simulink model "RobotControl1_640_480"  (R2015a)
settings: Solver=ode3  StartTime=0.0  StopTime=inf  FixedStep=1/30  RelTol=1e-3
undefined symbols (not defined in the file or in its folder): RGB24
libraries: xpcutilitieslib x31, slrtlib x8, AAxpcseriallibold x7, xpcobsoletelib x5, xpcvideousblib x3, dspstat3 x1, simulink x1
settings Model: SimulationMode=external  Creator=farbod  LastModifiedBy=sd0016
settings SolverCC: EnableConcurrentExecution=on
settings DataIOCC: SignalLoggingSaveFormat=ModelDataLogs
settings OptimizationCC: BlockReduction=off  OptimizeBlockIOStorage=off  BufferReuse=off  GlobalBufferReuse=off  ExpressionFolding=off  ExpressionDepthLimit=2147483647  LocalBlockOutputs=off
settings DebuggingCC: UnderspecifiedInitializationDetection=Classic  MergeDetectMultiDrivingBlocksExec=none  FcnCallInpInsideContextMsg=UseLocalSettings  StateNameClashWarn=warning
settings HardwareCC: ProdIntDivRoundTo=Zero  ProdEndianess=LittleEndian  ProdLongLongMode=on  ProdHWDeviceType=Generic->32-bit x86 compatible  TargetBitPerLong=64  TargetBitPerPointer=64  TargetIntDivRoundTo=Zero  TargetEndianess=LittleEndian  TargetWordSize=64  TargetHWDeviceType=Intel->x86-64
settings SFSimCC: SimParseCustomCode=off
settings RTWCC: SystemTargetFile=slrt.tlc  TemplateMakefile=slrt_default_tmf  Description=Simulink Real-Time  RTWVerbose=off  RTWCompilerOptimization=on
settings CodeAppCC: MaxIdLength=95
settings SimulinkRealTimeCC: GeneratePreprocessorConditionals=Disable all

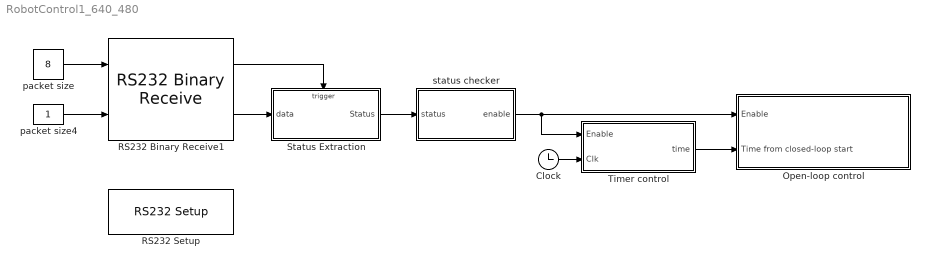
== system RobotControl1_640_480 ==
  Clock : Clock
  Open-loop control : Subsystem
  RS232 Binary Receive1 : AAxpcseriallibold/Obsolete/Binary Mode/RS232 Binary Receive  port=COM1  width=8  samptime=-1
  "RS232 Setup " : AAxpcseriallibold/Obsolete/RS232 Setup   port=COM1  baud=115200  dbits=8  sbits=1  parity=None  prot=None  sbuf=2048  rbuf=2048  initstruct=[]  termstruct=[]
  Status Extraction : Subsystem  TreatAsAtomicUnit=on
  Timer control : Subsystem
  packet size : Constant  Value=8
  packet size4 : Constant
  status checker : MATLAB Function  TreatAsAtomicUnit=on
  wires:
  status checker/1(enable) -> Open-loop control/1("Enable "), Timer control/1(Enable)
  Status Extraction/1(Status) -> status checker/1(status)
  RS232 Binary Receive1/2 -> Status Extraction/1(data)
  RS232 Binary Receive1/1 -> Status Extraction/Trigger
  packet size4/1 -> RS232 Binary Receive1/2
  packet size/1 -> RS232 Binary Receive1/1
  Timer control/1(time) -> Open-loop control/2(Time from closed-loop start)
  Clock/1 -> Timer control/2(Clk)

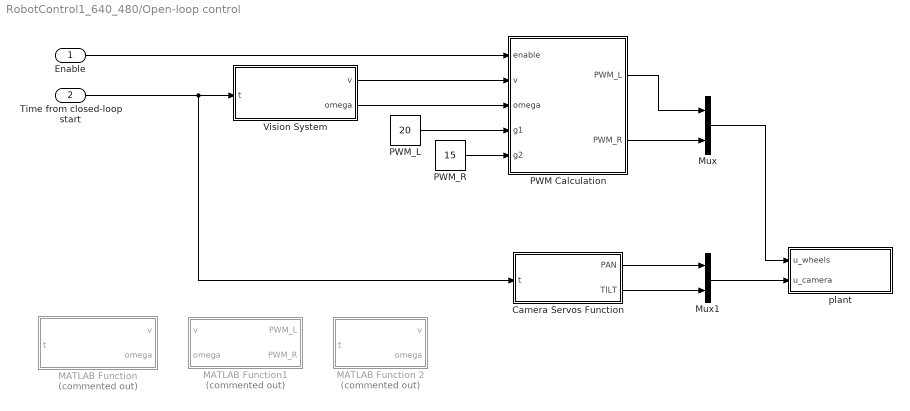
== system RobotControl1_640_480/Open-loop control ==
  "Enable " : Inport
  Time from closed-loop start : Inport  Port=2
  " MATLAB Function1" : MATLAB Function  Commented=on  TreatAsAtomicUnit=on
  Camera Servos Function : MATLAB Function  TreatAsAtomicUnit=on
  MATLAB Function : MATLAB Function  Commented=on  TreatAsAtomicUnit=on
  MATLAB Function 2 : MATLAB Function  Commented=on  TreatAsAtomicUnit=on
  Mux : Mux  Inputs=2
  Mux1 : Mux  Inputs=2
  PWM Calculation : MATLAB Function  TreatAsAtomicUnit=on
  PWM_L : Constant  Value=20
  PWM_R : Constant  Value=15
  Vision System : Subsystem
  plant : Subsystem
  wires:
  Mux/1 -> plant/1(u_wheels)
  Camera Servos Function/1(PAN) -> Mux1/1
  Camera Servos Function/2(TILT) -> Mux1/2
  Mux1/1 -> plant/2(u_camera)
  PWM Calculation/2(PWM_R) -> Mux/2
  "Enable "/1 -> PWM Calculation/1(enable)
  PWM Calculation/1(PWM_L) -> Mux/1
  Time from closed-loop start/1 -> Camera Servos Function/1(t), Vision System/1(t)
  Vision System/1(v) -> PWM Calculation/2(v)
  Vision System/2(omega) -> PWM Calculation/3(omega)
  PWM_L/1 -> PWM Calculation/4(g1)
  PWM_R/1 -> PWM Calculation/5(g2)

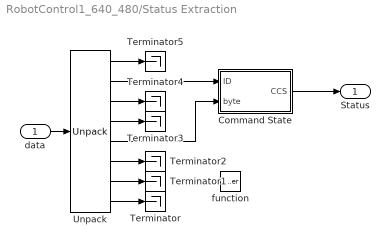
== system RobotControl1_640_480/Status Extraction ==
  data : Inport
  function : TriggerPort  TriggerType=function-call  OutputDataType=int8
  Command State : MATLAB Function  TreatAsAtomicUnit=on
  Terminator{,1..5} (6 alike) : Terminator
  Unpack : xpcobsoletelib/Utilities/Unpack   dimensions={1,1,1,1,1,1,1,1}  datatypes={'uint8','uint8','uint8','uint8','uint8','uint8','uint8','uint8'}  byteAlign=1
  Status : Outport
  wires:
  data/1 -> Unpack/1
  Command State/1(CCS) -> Status/1
  Unpack/5 -> Command State/2(byte)
  Unpack/2 -> Command State/1(ID)
  Unpack/8 -> Terminator/1
  Unpack/1 -> Terminator5/1
  Unpack/3 -> Terminator4/1
  Unpack/4 -> Terminator3/1
  Unpack/6 -> Terminator2/1
  Unpack/7 -> Terminator1/1

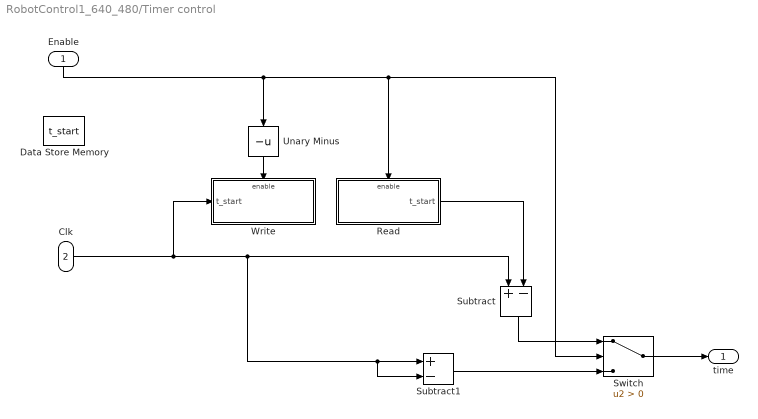
== system RobotControl1_640_480/Timer control ==
  Enable : Inport
  Clk : Inport  Port=2
  Data Store Memory : DataStoreMemory  DataStoreName=t_start  ReadBeforeWriteMsg=warning  WriteAfterWriteMsg=warning  WriteAfterReadMsg=warning
  Read : Subsystem  TreatAsAtomicUnit=on
  Subtract : Sum  Inputs=+-
  Subtract1 : Sum  Inputs=+-
  Switch : Switch  Criteria=u2 > Threshold
  Unary Minus : UnaryMinus
  Write : Subsystem  TreatAsAtomicUnit=on
  time : Outport
  wires:
  Read/1(t_start) -> Subtract/2
  Clk/1 -> Write/1(t_start), Subtract1/2, Subtract1/1, Subtract/1
  Unary Minus/1 -> Write/Enable
  Enable/1 -> Unary Minus/1, Read/Enable, Switch/2
  Switch/1 -> time/1
  Subtract/1 -> Switch/1
  Subtract1/1 -> Switch/3

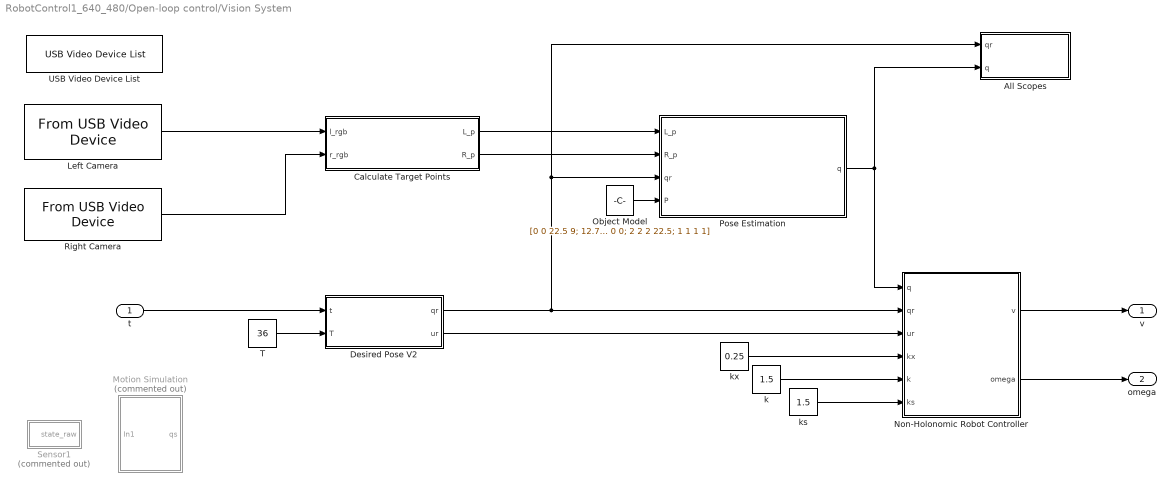
== system RobotControl1_640_480/Open-loop control/Vision System ==
  t : Inport
  All Scopes : Subsystem
  Calculate Target Points : MATLAB Function  TreatAsAtomicUnit=on
  Desired Pose V2 : MATLAB Function  TreatAsAtomicUnit=on
  Left Camera : xpcvideousblib/From USB Video Device  sconf=<Select a configuration>  paddr=1.0  iwidth=640  iheight=480  fint=1/30  ffmt=Uncompressed  cfmt=RGB24 (8:8:8)  isig=One multidimensional signal  trigger=off  status=off  updateBlock=1
  Motion Simulation : Subsystem  Commented=on
  Non-Holonomic Robot Controller : MATLAB Function  TreatAsAtomicUnit=on
  Object Model : Constant  Value=[0 0 22.5 9; 12.75 -12.75 0 0; 2 2 2 22.5; 1 1 1 1]
  Pose Estimation : MATLAB Function  TreatAsAtomicUnit=on
  Right Camera : xpcvideousblib/From USB Video Device  sconf=<Select a configuration>  paddr=1.3  iwidth=640  iheight=480  fint=1/30  ffmt=Uncompressed  cfmt=RGB24 (8:8:8)  isig=One multidimensional signal  trigger=off  status=off  updateBlock=1
  Sensor1 : Subsystem  Commented=on
  T : Constant  Value=36
  USB Video Device List : xpcvideousblib/USB Video Device List  usb_search=on  ShowInLibBrowser=0
  k : Constant  Value=1.5
  ks : Constant  Value=1.5
  kx : Constant  Value=0.25
  v : Outport
  omega : Outport  Port=2
  wires:
  Non-Holonomic Robot Controller/1(v) -> v/1
  Non-Holonomic Robot Controller/2(omega) -> omega/1
  Object Model/1 -> Pose Estimation/4(P)
  Left Camera/1 -> Calculate Target Points/1(l_rgb)
  Right Camera/1 -> Calculate Target Points/2(r_rgb)
  Calculate Target Points/1(L_p) -> Pose Estimation/1(L_p)
  Calculate Target Points/2(R_p) -> Pose Estimation/2(R_p)
  Desired Pose V2/1(qr) -> Pose Estimation/3(qr), All Scopes/1(qr), Non-Holonomic Robot Controller/2(qr)
  Desired Pose V2/2(ur) -> Non-Holonomic Robot Controller/3(ur)
  k/1 -> Non-Holonomic Robot Controller/5(k)
  kx/1 -> Non-Holonomic Robot Controller/4(kx)
  ks/1 -> Non-Holonomic Robot Controller/6(ks)
  T/1 -> Desired Pose V2/2(T)
  t/1 -> Desired Pose V2/1(t)
  Pose Estimation/1(q) -> All Scopes/2(q), Non-Holonomic Robot Controller/1(q)

== system RobotControl1_640_480/Open-loop control/plant ==
  u_wheels : Inport
  u_camera : Inport  Port=2
  Demux : Demux  Outputs=2
  Demux1 : Demux  Outputs=2
  Send Serial Packet to Servo Controller And recieve status message from SSC : Subsystem  TreatAsAtomicUnit=on
  Servo1 : Constant  Value=1500  OutDataTypeStr=uint16
  pulse transformer camera : MATLAB Function  TreatAsAtomicUnit=on
  pulse transformer1 : MATLAB Function  TreatAsAtomicUnit=on
  wires:
  Servo1/1 -> Send Serial Packet to Servo Controller And recieve status message from SSC/6(Servo6), Send Serial Packet to Servo Controller And recieve status message from SSC/8(Servo8), Send Serial Packet to Servo Controller And recieve status message from SSC/4(Servo4), Send Serial Packet to Servo Controller And recieve status message from SSC/1(Servo1)
  u_wheels/1 -> Demux/1
  Demux/1 -> pulse transformer1/1(Left_PWM_I)
  Demux/2 -> pulse transformer1/2(Right_PWM_I)
  u_camera/1 -> Demux1/1
  pulse transformer1/1(Left_PWM) -> Send Serial Packet to Servo Controller And recieve status message from SSC/2(Left)
  pulse transformer1/2(Right_PWM) -> Send Serial Packet to Servo Controller And recieve status message from SSC/3(Right)
  Demux1/1 -> pulse transformer camera/1(PAN)
  Demux1/2 -> pulse transformer camera/2(TILT)
  pulse transformer camera/1(PAN_O) -> Send Serial Packet to Servo Controller And recieve status message from SSC/5(Pan)
  pulse transformer camera/2(TILT_O) -> Send Serial Packet to Servo Controller And recieve status message from SSC/7(Tilt)

== system RobotControl1_640_480/Timer control/Read ==
  Enable : EnablePort
  Data Store Read : DataStoreRead  DataStoreName=t_start
  t_start : Outport
  wires:
  Data Store Read/1 -> t_start/1

== system RobotControl1_640_480/Timer control/Write ==
  t_start : Inport
  Enable : EnablePort
  Data Store Write : DataStoreWrite  DataStoreName=t_start
  wires:
  t_start/1 -> Data Store Write/1

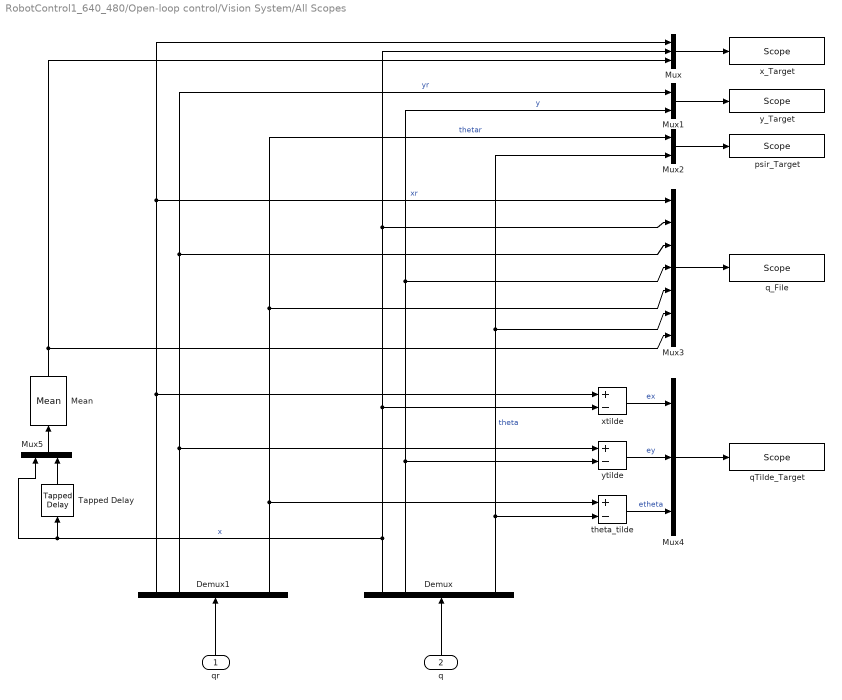
== system RobotControl1_640_480/Open-loop control/Vision System/All Scopes ==
  qr : Inport
  q : Inport  Port=2
  Demux : Demux  Outputs=6
  Demux1 : Demux  Outputs=6
  Mean : dspstat3/Mean  run=off  reset_popup=None  InputProcessing=Columns as channels (frame based)  directionMode=Each column  dimension=1  treatSBRowAsCol=off  roiEnable=off  roiType=Rectangles  roiPortion=Entire ROI  roiOutput=Individual statistics for each ROI  roiFlag=off  outputDataTypeStr=Inherit: Same as accumulator  outputLastDataTypeStr=Inherit: Same as accumulator  outputMin=[]  outputMax=[]  roundingMode=Floor  overflowMode=off
  Mux : Mux  Inputs=3
  Mux1 : Mux  Inputs=2
  Mux2 : Mux  Inputs=2
  Mux3 : Mux  Inputs=7
  Mux4 : Mux  Inputs=3
  Mux5 : Mux  Inputs=2
  Tapped Delay : simulink/Discrete/Tapped Delay  vinit=[0 0]  samptime=-1  NumDelays=2  DelayOrder=Oldest  includeCurrent=off
  "psir_Target " : slrtlib/Displays and Logging/Scope   scopeno=6  scopetype=Target  autostart=on  viewmode=Graphical rolling  formatstr='%15.6f'  grid=on  ylimits=[-3, 3]  nosamples=1000  noprepostsamples=0  interleave=1  triggermode=FreeRun  triggersignal=1  trigsignalfromport=off  triggerlevel=0.0  triggerslope=Either  triggerscope=1  triggersample=0  filename=data.dat  mode=Lazy  writesize=512  autorestart=off  dynamicfilemode=off  maxwritefilesize=512*1024^2
  qTilde_Target : slrtlib/Displays and Logging/Scope   scopeno=3  scopetype=Target  autostart=on  viewmode=Numerical  formatstr='%15.6f'  grid=on  ylimits=[0,0]  nosamples=3  noprepostsamples=0  interleave=1  triggermode=FreeRun  triggersignal=1  trigsignalfromport=off  triggerlevel=0.0  triggerslope=Either  triggerscope=1  triggersample=0  filename=data.dat  mode=Lazy  writesize=512  autorestart=off  dynamicfilemode=off  maxwritefilesize=512*1024^2
  q_File : slrtlib/Displays and Logging/Scope   scopeno=2  scopetype=File  autostart=on  viewmode=Graphical redraw  formatstr='%15.6f'  grid=on  ylimits=[0,0]  nosamples=6000  noprepostsamples=0  interleave=1  triggermode=FreeRun  triggersignal=1  trigsignalfromport=off  triggerlevel=0.0  triggerslope=Either  triggerscope=1  triggersample=0  filename=q.dat  mode=Lazy  writesize=512  autorestart=off  dynamicfilemode=off  maxwritefilesize=512*1024^2
  theta_tilde : Sum  Inputs=+-
  "x_Target " : slrtlib/Displays and Logging/Scope   scopeno=1  scopetype=Target  autostart=on  viewmode=Graphical rolling  formatstr='%15.6f'  grid=on  ylimits=[-4.5, 0.5]  nosamples=1000  noprepostsamples=0  interleave=1  triggermode=FreeRun  triggersignal=1  trigsignalfromport=off  triggerlevel=0.0  triggerslope=Either  triggerscope=1  triggersample=0  filename=data.dat  mode=Lazy  writesize=512  autorestart=off  dynamicfilemode=off  maxwritefilesize=512*1024^2
  xtilde : Sum  Inputs=+-
  y_Target : slrtlib/Displays and Logging/Scope   scopeno=4  scopetype=Target  autostart=on  viewmode=Graphical rolling  formatstr='%15.6f'  grid=on  ylimits=[-2,2]  nosamples=1000  noprepostsamples=0  interleave=1  triggermode=FreeRun  triggersignal=1  trigsignalfromport=off  triggerlevel=0.0  triggerslope=Either  triggerscope=1  triggersample=0  filename=data.dat  mode=Lazy  writesize=512  autorestart=off  dynamicfilemode=off  maxwritefilesize=512*1024^2
  ytilde : Sum  Inputs=+-
  wires:
  q/1 -> Demux/1
  Demux1/1 -> xtilde/1, Mux/1, Mux3/1  "xr"
  Demux1/2 -> ytilde/1, Mux1/1, Mux3/3  "yr"
  Mux3/1 -> q_File/1
  qr/1 -> Demux1/1
  Mux1/1 -> y_Target/1
  Mux/1 -> "x_Target "/1
  Mux2/1 -> "psir_Target "/1
  Demux/6 -> theta_tilde/2, Mux3/6, Mux2/2  "theta"
  Demux1/6 -> theta_tilde/1, Mux2/1, Mux3/5  "thetar"
  Demux/2 -> ytilde/2, Mux3/4, Mux1/2  "y"
  Demux/1 -> Mux5/1, Tapped Delay/1, xtilde/2, Mux3/2, Mux/2  "x"
  theta_tilde/1 -> Mux4/3  "etheta"
  ytilde/1 -> Mux4/2  "ey"
  xtilde/1 -> Mux4/1  "ex"
  Mux4/1 -> qTilde_Target/1
  Tapped Delay/1 -> Mux5/2
  Mean/1 -> Mux/3, Mux3/7
  Mux5/1 -> Mean/1

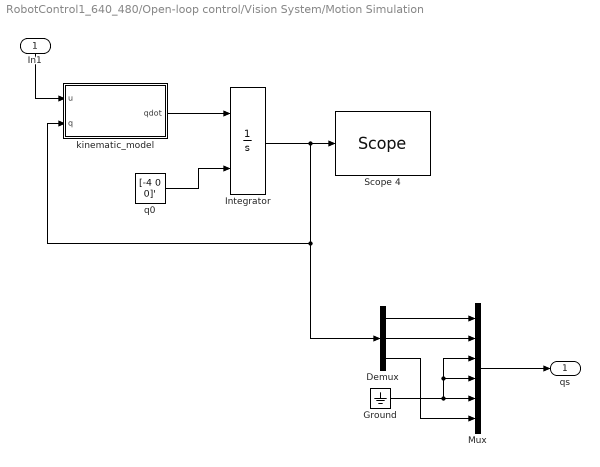
== system RobotControl1_640_480/Open-loop control/Vision System/Motion Simulation ==
  In1 : Inport
  Demux : Demux  Outputs=3
  Ground : Ground
  Integrator : Integrator  InitialConditionSource=external
  Mux : Mux  Inputs=6
  Scope 4 : slrtlib/Displays and Logging/Scope   scopeno=30  scopetype=File  autostart=on  viewmode=Graphical rolling  formatstr='%15.6f'  grid=on  ylimits=[0,0]  nosamples=250  noprepostsamples=0  interleave=1  triggermode=FreeRun  triggersignal=1  trigsignalfromport=off  triggerlevel=0.0  triggerslope=Either  triggerscope=1  triggersample=0  filename=data.dat  mode=Lazy  writesize=512  autorestart=off  dynamicfilemode=off  maxwritefilesize=512*1024^2
  kinematic_model : MATLAB Function  TreatAsAtomicUnit=on
  q0 : Constant  Value=[-4 0 0]'
  qs : Outport
  wires:
  kinematic_model/1(qdot) -> Integrator/1
  In1/1 -> kinematic_model/1(u)
  Integrator/1 -> Demux/1, kinematic_model/2(q), Scope 4/1
  q0/1 -> Integrator/2
  Mux/1 -> qs/1
  Demux/1 -> Mux/1
  Demux/2 -> Mux/2
  Demux/3 -> Mux/6
  Ground/1 -> Mux/5, Mux/3, Mux/4

== system RobotControl1_640_480/Open-loop control/Vision System/Sensor1 ==
  Add : Sum  Inputs=+-
  Clock2 : Clock
  Command State : MATLAB Function  TreatAsAtomicUnit=on
  IMU Trigger : Subsystem
  Read_Filter_ConvertTo2D : Subsystem
  delay : Constant
  state_raw : Outport
  wires:
  Clock2/1 -> Add/1, Command State/1(clock)
  Read_Filter_ConvertTo2D/1(state_raw) -> state_raw/1
  delay/1 -> Add/2
  Add/1 -> Read_Filter_ConvertTo2D/Enable
  Command State/1(Status) -> IMU Trigger/Enable

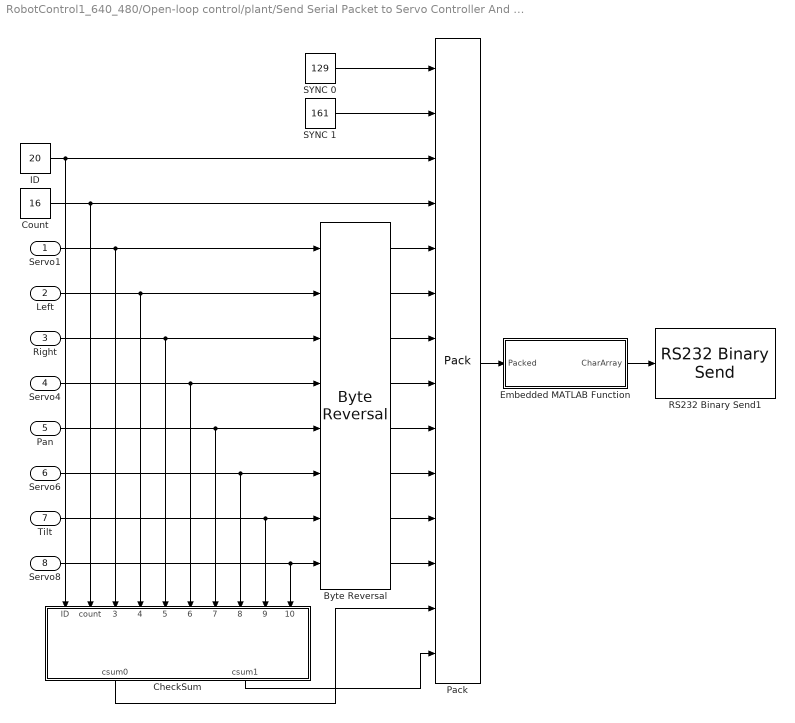
== system RobotControl1_640_480/Open-loop control/plant/Send Serial Packet to Servo Controller And recieve status message from SSC ==
  Servo1 : Inport  OutDataTypeStr=uint16
  Left : Inport  Port=2  OutDataTypeStr=uint16
  Right : Inport  Port=3  OutDataTypeStr=uint16
  Servo4 : Inport  Port=4  OutDataTypeStr=uint16
  Pan : Inport  Port=5  OutDataTypeStr=uint16
  Servo6 : Inport  Port=6  OutDataTypeStr=uint16
  Tilt : Inport  Port=7  OutDataTypeStr=uint16
  Servo8 : Inport  Port=8  OutDataTypeStr=uint16
  Byte Reversal : xpcutilitieslib/Byte Reversal   numInp=8
  CheckSum : MATLAB Function  TreatAsAtomicUnit=on
  Count : Constant  Value=16  OutDataTypeStr=uint8
  Embedded MATLAB Function : MATLAB Function  TreatAsAtomicUnit=on
  ID : Constant  Value=20  OutDataTypeStr=uint8
  Pack : xpcobsoletelib/Utilities/Pack   datatypes={'uint8','uint8','uint8','uint8','uint16','uint16','uint16','uint16','uint16','uint16','uint16','uint16','uint8','uint8'}  byteAlign=1
  RS232 Binary Send1 : AAxpcseriallibold/Obsolete/Binary Mode/RS232 Binary Send  port=COM1  width=22  samptime=-1
  SYNC 0 : Constant  Value=129  OutDataTypeStr=uint8
  SYNC 1 : Constant  Value=161  OutDataTypeStr=uint8
  wires:
  SYNC 0/1 -> Pack/1
  SYNC 1/1 -> Pack/2
  ID/1 -> Pack/3, CheckSum/1(ID)
  Count/1 -> Pack/4, CheckSum/2(count)
  Byte Reversal/2 -> Pack/6
  Byte Reversal/1 -> Pack/5
  Byte Reversal/3 -> Pack/7
  Byte Reversal/4 -> Pack/8
  Byte Reversal/5 -> Pack/9
  Byte Reversal/6 -> Pack/10
  Byte Reversal/7 -> Pack/11
  Byte Reversal/8 -> Pack/12
  CheckSum/2(csum1) -> Pack/14
  CheckSum/1(csum0) -> Pack/13
  Servo8/1 -> Byte Reversal/8, CheckSum/10(servo8)
  Tilt/1 -> Byte Reversal/7, CheckSum/9(servo7)
  Servo6/1 -> Byte Reversal/6, CheckSum/8(servo6)
  Pan/1 -> Byte Reversal/5, CheckSum/7(servo5)
  Servo4/1 -> Byte Reversal/4, CheckSum/6(servo4)
  Right/1 -> Byte Reversal/3, CheckSum/5(servo3)
  Left/1 -> Byte Reversal/2, CheckSum/4(servo2)
  Servo1/1 -> Byte Reversal/1, CheckSum/3(servo1)
  Pack/1 -> Embedded MATLAB Function/1(Packed)
  Embedded MATLAB Function/1(CharArray) -> RS232 Binary Send1/1

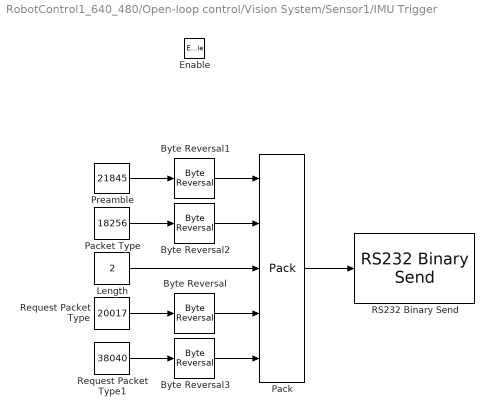
== system RobotControl1_640_480/Open-loop control/Vision System/Sensor1/IMU Trigger ==
  Enable : EnablePort  PropagateVarSize=During execution
  Byte Reversal{,1..3} (4 alike) : xpcutilitieslib/Byte Reversal   numInp=1
  Length : Constant  Value=2  OutDataTypeStr=uint8
  Pack : xpcobsoletelib/Utilities/Pack   datatypes={'uint16','uint16','uint8','uint16','uint16'}  byteAlign=1
  Packet Type : Constant  Value=18256  OutDataTypeStr=uint16
  Preamble : Constant  Value=21845  OutDataTypeStr=uint16
  RS232 Binary Send : AAxpcseriallibold/Obsolete/Binary Mode/RS232 Binary Send  port=COM2  width=9  samptime=-1
  Request Packet Type : Constant  Value=20017  OutDataTypeStr=uint16
  Request Packet Type1 : Constant  Value=38040  OutDataTypeStr=uint16
  wires:
  Pack/1 -> RS232 Binary Send/1
  Preamble/1 -> Byte Reversal1/1
  Packet Type/1 -> Byte Reversal2/1
  Length/1 -> Pack/3
  Request Packet Type/1 -> Byte Reversal/1
  Request Packet Type1/1 -> Byte Reversal3/1
  Byte Reversal/1 -> Pack/4
  Byte Reversal1/1 -> Pack/1
  Byte Reversal2/1 -> Pack/2
  Byte Reversal3/1 -> Pack/5

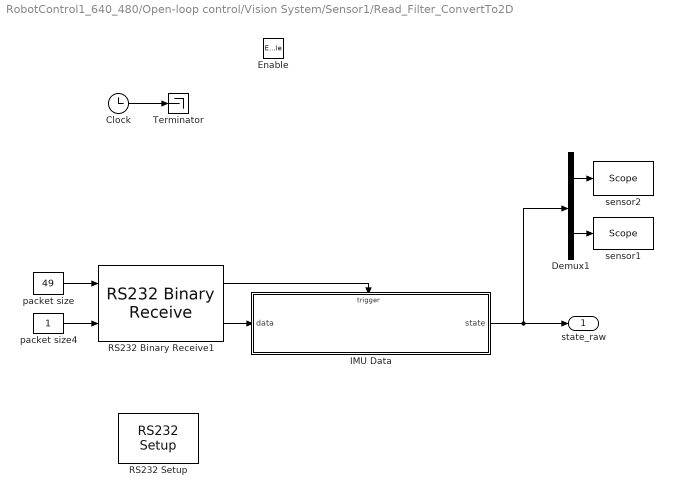
== system RobotControl1_640_480/Open-loop control/Vision System/Sensor1/Read_Filter_ConvertTo2D ==
  Enable : EnablePort  PropagateVarSize=During execution
  Clock : Clock
  Demux1 : Demux  Outputs=2
  IMU Data : Subsystem  TreatAsAtomicUnit=on
  RS232 Binary Receive1 : AAxpcseriallibold/Obsolete/Binary Mode/RS232 Binary Receive  port=COM2  width=49  samptime=-1
  "RS232 Setup " : AAxpcseriallibold/Obsolete/RS232 Setup   port=COM2  baud=57600  dbits=8  sbits=1  parity=None  prot=None  sbuf=1024  rbuf=1024  initstruct=[]  termstruct=[]
  Terminator : Terminator
  packet size : Constant  Value=49
  packet size4 : Constant
  sensor1 : slrtlib/Displays and Logging/Scope   scopeno=4  scopetype=File  autostart=on  viewmode=Graphical rolling  formatstr='%15.6f'  grid=on  ylimits=[-10,50]  nosamples=3000  noprepostsamples=0  interleave=1  triggermode=FreeRun  triggersignal=1  trigsignalfromport=off  triggerlevel=0.0  triggerslope=Either  triggerscope=1  triggersample=0  filename=1sens15.dat  mode=Commit  writesize=512  autorestart=on  dynamicfilemode=off  maxwritefilesize=512*1024^2
  sensor2 : slrtlib/Displays and Logging/Scope   scopeno=6  scopetype=File  autostart=on  viewmode=Graphical rolling  formatstr='%15.6f'  grid=on  ylimits=[-10,50]  nosamples=3000  noprepostsamples=0  interleave=1  triggermode=FreeRun  triggersignal=1  trigsignalfromport=off  triggerlevel=0.0  triggerslope=Either  triggerscope=1  triggersample=0  filename=1sens16.dat  mode=Commit  writesize=512  autorestart=on  dynamicfilemode=off  maxwritefilesize=512*1024^2
  state_raw : Outport
  wires:
  Demux1/2 -> sensor1/1
  Demux1/1 -> sensor2/1
  Clock/1 -> Terminator/1
  packet size/1 -> RS232 Binary Receive1/1
  packet size4/1 -> RS232 Binary Receive1/2
  IMU Data/1(state) -> Demux1/1, state_raw/1
  RS232 Binary Receive1/2 -> IMU Data/1(data)
  RS232 Binary Receive1/1 -> IMU Data/Trigger

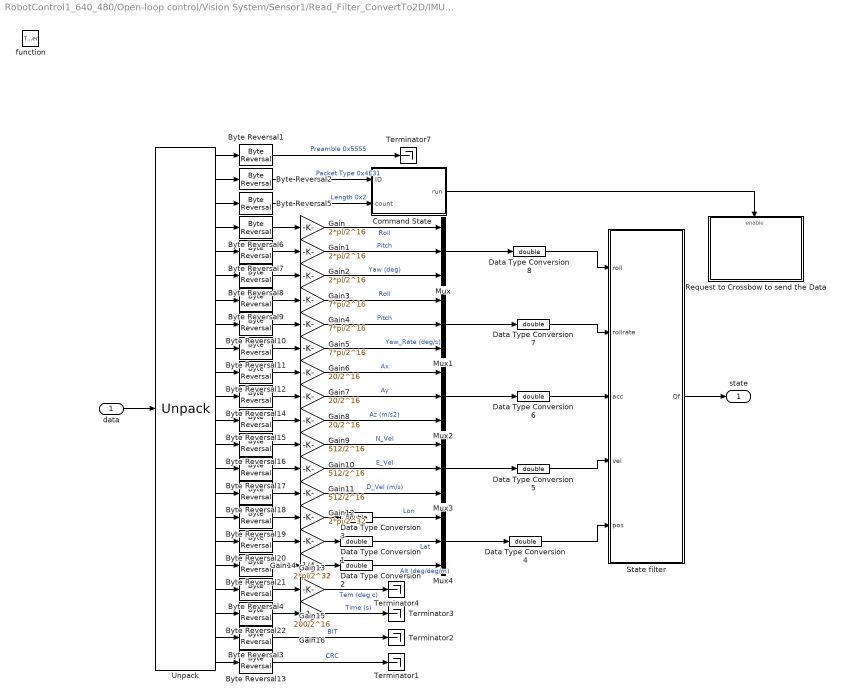
== system RobotControl1_640_480/Open-loop control/Vision System/Sensor1/Read_Filter_ConvertTo2D/IMU Data ==
  data : Inport
  function : TriggerPort  TriggerType=function-call  OutputDataType=int8
  Byte Reversal{1..22} (22 alike) : xpcutilitieslib/Byte Reversal   numInp=1
  Command State : MATLAB Function  TreatAsAtomicUnit=on
  Data Type Conversion{1..8} (8 alike) : DataTypeConversion  OutDataTypeStr=double
  Gain : Gain  Gain=2*pi/2^16
  Gain1 : Gain  Gain=2*pi/2^16
  Gain10 : Gain  Gain=512/2^16
  Gain11 : Gain  Gain=512/2^16
  Gain12 : Gain  Gain=2*pi/2^32
  Gain13 : Gain  Gain=2*pi/2^32
  Gain14 : Gain  Gain=1/4
  Gain15 : Gain  Gain=200/2^16
  Gain16 : Gain
  Gain2 : Gain  Gain=2*pi/2^16
  Gain3 : Gain  Gain=7*pi/2^16
  Gain4 : Gain  Gain=7*pi/2^16
  Gain5 : Gain  Gain=7*pi/2^16
  Gain6 : Gain  Gain=20/2^16
  Gain7 : Gain  Gain=20/2^16
  Gain8 : Gain  Gain=20/2^16
  Gain9 : Gain  Gain=512/2^16
  Mux{,1..4} (5 alike) : Mux  Inputs=3
  Request to Crossbow to send the Data : Subsystem
  State filter : MATLAB Function  TreatAsAtomicUnit=on
  Terminator{1..4,7} (5 alike) : Terminator
  Unpack : xpcobsoletelib/Utilities/Unpack   dimensions={1,1,1,1,1,1,1,1,1,1,1,1,1,1,1,1,1,1,1,1,1,1}  datatypes={'uint16','uint16','uint8','int16','int16','int16','int16','int16','int16','int16','int16','int16','int16','int16','int16','int32','int32','int16','int16','uint32','uint16','uint16'}  byteAlign=1
  state : Outport
  wires:
  data/1 -> Unpack/1
  Unpack/1 -> Byte Reversal1/1
  Unpack/2 -> Byte Reversal2/1
  Unpack/3 -> Byte Reversal5/1
  Unpack/4 -> Byte Reversal6/1
  Unpack/5 -> Byte Reversal7/1
  Unpack/6 -> Byte Reversal8/1
  Unpack/7 -> Byte Reversal9/1
  Unpack/8 -> Byte Reversal10/1
  Byte Reversal1/1 -> Terminator7/1  "Preamble 0x5555"
  Byte Reversal2/1 -> Command State/1(ID)  "Packet Type 0x4E31"
  Command State/1(run) -> Request to Crossbow to send the Data/Enable
  Unpack/21 -> Byte Reversal3/1
  Unpack/19 -> Byte Reversal4/1
  Byte Reversal5/1 -> Command State/2(count)  "Length 0x2"
  Byte Reversal9/1 -> Gain3/1
  Byte Reversal10/1 -> Gain4/1
  Byte Reversal6/1 -> Gain/1
  Byte Reversal7/1 -> Gain1/1
  Byte Reversal8/1 -> Gain2/1
  Gain/1 -> Mux/1  "Roll"
  Gain1/1 -> Mux/2  "Pitch"
  Gain2/1 -> Mux/3  "Yaw (deg)"
  Gain3/1 -> Mux1/1  "Roll"
  Gain4/1 -> Mux1/2  "Pitch"
  Unpack/9 -> Byte Reversal11/1
  Byte Reversal11/1 -> Gain5/1
  Gain5/1 -> Mux1/3  "Yaw_Rate (deg/s)"
  Gain6/1 -> Mux2/1  "Ax"
  Byte Reversal12/1 -> Gain6/1
  Unpack/10 -> Byte Reversal12/1
  Mux/1 -> Data Type Conversion8/1
  Unpack/22 -> Byte Reversal13/1
  Byte Reversal3/1 -> Terminator2/1  "BIT"
  Byte Reversal13/1 -> Terminator1/1  "CRC"
  Unpack/20 -> Byte Reversal22/1
  Mux1/1 -> Data Type Conversion7/1
  Mux2/1 -> Data Type Conversion6/1
  Byte Reversal14/1 -> Gain7/1
  Byte Reversal15/1 -> Gain8/1
  Unpack/11 -> Byte Reversal14/1
  Unpack/12 -> Byte Reversal15/1
  Gain7/1 -> Mux2/2  "Ay"
  Gain8/1 -> Mux2/3  "Az (m/s2)"
  Mux3/1 -> Data Type Conversion5/1
  Unpack/13 -> Byte Reversal16/1
  Byte Reversal16/1 -> Gain9/1
  Byte Reversal17/1 -> Gain10/1
  Byte Reversal18/1 -> Gain11/1
  Unpack/14 -> Byte Reversal17/1
  Unpack/15 -> Byte Reversal18/1
  Gain9/1 -> Mux3/1  "N_Vel"
  Gain10/1 -> Mux3/2  "E_Vel"
  Gain11/1 -> Mux3/3  "D_Vel (m/s)"
  Unpack/16 -> Byte Reversal19/1
  Unpack/17 -> Byte Reversal20/1
  Unpack/18 -> Byte Reversal21/1
  Byte Reversal20/1 -> Gain13/1
  Byte Reversal19/1 -> Gain12/1
  Mux4/1 -> Data Type Conversion4/1
  Gain12/1 -> Data Type Conversion3/1
  Gain13/1 -> Data Type Conversion1/1
  Gain14/1 -> Data Type Conversion2/1
  Byte Reversal21/1 -> Gain14/1
  Byte Reversal22/1 -> Gain16/1
  Byte Reversal4/1 -> Gain15/1
  Gain15/1 -> Terminator4/1  "Tem (deg c)"
  Gain16/1 -> Terminator3/1  "Time (s)"
  Data Type Conversion2/1 -> Mux4/3  "Alt (deg/deg/m)"
  Data Type Conversion1/1 -> Mux4/2  "Lat"
  Data Type Conversion3/1 -> Mux4/1  "Lon"
  State filter/1(Qf) -> state/1
  Data Type Conversion4/1 -> State filter/5(pos)
  Data Type Conversion5/1 -> State filter/4(vel)
  Data Type Conversion6/1 -> State filter/3(acc)
  Data Type Conversion7/1 -> State filter/2(rollrate)
  Data Type Conversion8/1 -> State filter/1(roll)

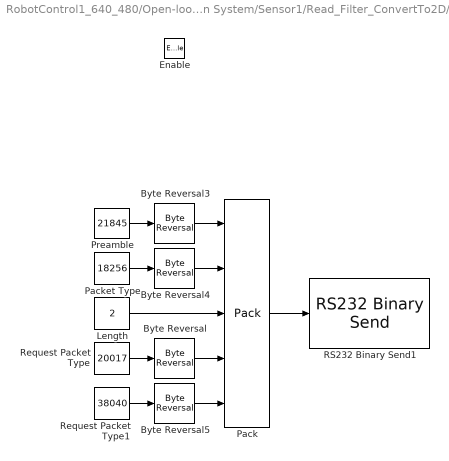
== system RobotControl1_640_480/Open-loop control/Vision System/Sensor1/Read_Filter_ConvertTo2D/IMU Data/Request to Crossbow to send the Data ==
  Enable : EnablePort  PropagateVarSize=During execution
  Byte Reversal{,3..5} (4 alike) : xpcutilitieslib/Byte Reversal   numInp=1
  Length : Constant  Value=2  OutDataTypeStr=uint8
  Pack : xpcobsoletelib/Utilities/Pack   datatypes={'uint16','uint16','uint8','uint16','uint16'}  byteAlign=1
  Packet Type : Constant  Value=18256  OutDataTypeStr=uint16
  Preamble : Constant  Value=21845  OutDataTypeStr=uint16
  RS232 Binary Send1 : AAxpcseriallibold/Obsolete/Binary Mode/RS232 Binary Send  port=COM2  width=9  samptime=-1
  Request Packet Type : Constant  Value=20017  OutDataTypeStr=uint16
  Request Packet Type1 : Constant  Value=38040  OutDataTypeStr=uint16
  wires:
  Pack/1 -> RS232 Binary Send1/1
  Preamble/1 -> Byte Reversal3/1
  Packet Type/1 -> Byte Reversal4/1
  Length/1 -> Pack/3
  Request Packet Type/1 -> Byte Reversal/1
  Request Packet Type1/1 -> Byte Reversal5/1
  Byte Reversal/1 -> Pack/4
  Byte Reversal3/1 -> Pack/1
  Byte Reversal4/1 -> Pack/2
  Byte Reversal5/1 -> Pack/5

== matlab function RobotControl1_640_480/Open-loop control/MATLAB Function 2 ==
  data: t input; v output; omega output
function [v,omega] = fcn(t)
%#codegen

tau = 10;

v0 = 0.9;
omega0 = 0.5;

tshift = 1;

v = v0*sin(2*pi*t/tau);
omega = omega0*sin(2*pi*(t-tshift)/tau);

== matlab function RobotControl1_640_480/Open-loop control/Vision System/Non-Holonomic Robot Controller ==
  data: q input; qr input; ur input; kx input; k input; ks input; v output; omega output
function [v, omega] = controller(q,qr,ur,kx,k,ks)
% the controller
% u = [v omega]^T
% qtilde: posture error
% qr    : reference (desired) posture

%%----------Input Parametleri Duzenleniyor---------------------------------

u = zeros(2,1);

% for now
vr     = ur(1,1);
omegar = ur(2,1);

% According to the vision system: qtilde = q - qr, so
% q = qtilde + qr;

xr     = qr(1,1);
yr     = qr(2,1);
thetar = qr(6,1);

x     = q(1,1);
y     = q(2,1);
theta = q(6,1);

s = sin(theta);
c = cos(theta);

%% -------------------------Error Hesaplaniyor----------------------------
% Burada temelde 3 tane olan hata parametreleri 4 e cikariliyor. 
% theta parametresi es ve ec olarak iki ayri hata parametresine cevriliyor

% Eq.(4), third element!
etheta = thetar-theta;

% Local errors from Eq.(10)
ex = c*(xr - x) + s*(yr - y);
ey = -s*(xr - x) + c*(yr - y);

es = sin(thetar-theta);
ecos = cos(thetar-theta);

ec = ecos - 1;

%--------------------------------------------------------------------------
%% - u ya ulasabilmek icin ihtiyacimiz olanlar
% vb,omegab,vr,omegar: ilk ikisi hesaplaniyor son ikisi ur'den geliyor.
% k,kx,ks,a,n paper temel alinarak secilmis secilmis

% according to the paper
% k = 0.8; % k > 0
% kx = 0.2; % kx(t) > 0
% ks = 0.8; % ks(t) > 0
a = 3; % a > 2
n = 0; % n = -2, -1, 0, 1 or 2

% Eq.(18)
vb = kx*ex;
omegab = k*vr*ey*(1+ec/a)^2+ks*es*((1+ec/a)^2)^n;

v = (vr*cos(etheta)+vb); 
omega = omegar+omegab; % Eq.(6)

%buradaki u degeri controllerdan cikan ve sisteme giris olarak verilen u

% out = [xr x yr y ex vr omegab omegar];

== matlab function RobotControl1_640_480/Open-loop control/plant/Send Serial Packet to Servo Controller And recieve status message from SSC/CheckSum ==
  data: ID input; csum0 output; count input; servo1 input; servo2 input; csum1 output; servo3 input; servo4 input; servo5 input; servo6 input; servo7 input; servo8 input
function [csum0,csum1]= fcn(ID,count,servo1,servo2,servo3,servo4,servo5,servo6,servo7,servo8)
% The purpose of this function is to calculate the fletcher checksum values
% as defined in internet RFC 1145
% See page 11 of the Microbotics Servo Switch/Controller Users Manual for 
% more information

% break into bytes
servo1a=uint8(bitshift(servo1,-8)); servo1b=uint8(servo1-uint16(servo1a)*256);
servo2a=uint8(bitshift(servo2,-8)); servo2b=uint8(servo2-uint16(servo2a)*256);
servo3a=uint8(bitshift(servo3,-8)); servo3b=uint8(servo3-uint16(servo3a)*256);
servo4a=uint8(bitshift(servo4,-8)); servo4b=uint8(servo4-uint16(servo4a)*256);
servo5a=uint8(bitshift(servo5,-8)); servo5b=uint8(servo5-uint16(servo5a)*256);
servo6a=uint8(bitshift(servo6,-8)); servo6b=uint8(servo6-uint16(servo6a)*256);
servo7a=uint8(bitshift(servo7,-8)); servo7b=uint8(servo7-uint16(servo7a)*256);
servo8a=uint8(bitshift(servo8,-8)); servo8b=uint8(servo8-uint16(servo8a)*256);
byte=[ID, count, servo1a, servo1b, servo2a, servo2b, servo3a, servo3b, servo4a, servo4b, servo5a, servo5b, servo6a, servo6b, servo7a, servo7b, servo8a, servo8b];

cksum0=uint16(0);cksum1=uint16(0); % initialize to zero
for i=1:(count+2)
    cksum0=mod((cksum0+uint16(byte(i))),256);
    cksum1=mod((cksum1+cksum0),256);
end

csum0=uint8(cksum0); csum1=uint8(cksum1);

== matlab function RobotControl1_640_480/Open-loop control/ MATLAB Function1 ==
  data: v input; PWM_L output; omega input; PWM_R output
function [PWM_L,PWM_R] = fcn(v,omega)
%#codegen
v = -v;
omega = -omega;

T = 0.422;

vL = v -(T/2)*omega;
vR = v +(T/2)*omega;

vVec = [vL;vR];

aL = 3.8863614532;
bL = -0.0026808274;

aR = 3.2707294485;
bR = -0.0022447804;

A = [aL;aR];
B = [[bL,0];[0,bR]];

PWM = (B)\(vVec-A);

PWM_L = 1350;%PWM(1);
PWM_R = 1350;%PWM(2);

== matlab function RobotControl1_640_480/Open-loop control/Vision System/Sensor1/Command State ==
  data: clock input; Status output
function Status = fcn(clock)

% Initialization:

if clock == 0
    out = 1;
else
    out = 0;
end
Status = out;

== matlab function RobotControl1_640_480/Open-loop control/Vision System/Calculate Target Points ==
  settings: sampleTime=1/7.5
  data: l_rgb input; L_p output; r_rgb input; R_p output
function [L_p, R_p] = getCenter(l_rgb,r_rgb)

    %#codegen
    L_p=zeros(2,4);
    R_p=zeros(2,4);
    
    %input left image(l_rgb), right image(r_rgb), Pose target position 
    [m,~,~]=size(l_rgb);
    
    l_rgb1 = imcomplement(l_rgb);        % converts RGB to CMY color space 
    r_rgb1 = imcomplement(r_rgb);        % converts RGB to CMY color space 
    
    l_gray = 0.2989 * l_rgb1(:,:,1) + 0.5870 * l_rgb1(:,:,2) + 0.1140 * l_rgb1(:,:,3); % rgb2gray(rgb) ;convert rgb to grayscale 
    r_gray = 0.2989 * r_rgb1(:,:,1) + 0.5870 * r_rgb1(:,:,2) + 0.1140 * r_rgb1(:,:,3); % rgb2gray(rgb) ;convert rgb to grayscale
    
    l_rgb2 = l_rgb1(:,:,3)-l_gray;       % imsubtract(rgb1(:,:,3),gray)
    r_rgb2 = r_rgb1(:,:,3)-r_gray;       % imsubtract(rgb1(:,:,3),gray) 
        
    l_bw = l_rgb2 > 50;
    r_bw = r_rgb2 > 50;
    
    %finds yellow regions in image using BlobAnalysis.
    hblob = vision.BlobAnalysis;

    [l_area,l_center,~] = step(hblob, l_bw); % get [x y] is a centroid of region
    [r_area,r_center,~] = step(hblob, r_bw); % get [x y] is a centroid of region
    
    [~, indL] = sort(l_area,'descend');
    [~, indR] = sort(r_area,'descend');
    
    if(length(indL) >= 4 && length(indR) >= 4)
        L_p = l_center(indL(1:4),[1 2])';
        R_p = r_center(indR(1:4),[1 2])';

        L_p = orderPoints(L_p,m); 
        R_p = orderPoints(R_p,m);
    end
end

== matlab function RobotControl1_640_480/Open-loop control/Vision System/Pose Estimation ==
  data: L_p input; R_p input; qr input; q output; P input
function q = estimatePose(L_p,R_p,qr,P)
%#codegen

%Desired Robot Pose for current step qr()
robotPoseDes.x = qr(1);
robotPoseDes.y = qr(2);
robotPoseDes.z = qr(3);
robotPoseDes.phi = qr(4);
robotPoseDes.theta = qr(5);
robotPoseDes.psi = qr(6);

%Transform target points from I space into Desired Robot Space
world2robotDes = inv(EulerTrans(robotPoseDes));
S_PDes = world2robotDes*P;

%Calculate the error parameters for current step
errParams = mirage(L_p,R_p,S_PDes);

poseErrorMat = eye(4,4);
poseErrorMat(1:3,:) = reshape(errParams,3,4);

world2robot = poseErrorMat*world2robotDes;

robotPoseEst = calculatePose(world2robot);

q = [-robotPoseEst.x/100 -robotPoseEst.y/100 -robotPoseEst.z/100 -robotPoseEst.phi   -robotPoseEst.theta -robotPoseEst.psi]';

%Temporary Code
if(abs(q(1) - qr(1)) > 0.8)
    q(1) = qr(1);
    q(2) = qr(2);
end

if(abs(q(6) - qr(6)) > 0.8)
    q(6) = qr(6);
end

% qtilde = [ -robotPoseEst.x/100  - robotPoseDes.x;
%            -robotPoseEst.y/100  - robotPoseDes.y;
%            -robotPoseEst.z/100  - robotPoseDes.z;
%            -robotPoseEst.phi  - robotPoseDes.phi;
%            -robotPoseEst.theta  - robotPoseDes.theta;
%            -robotPoseEst.psi  - robotPoseDes.psi;];
       
end

== matlab function RobotControl1_640_480/Open-loop control/Vision System/Desired Pose V2 ==
  data: t input; T input; qr output; ur output
function [qr, ur] = desired(t,T)
%#codegen

    x0 = 4;
    xc = 0.9;
%     T = 36;
    
    if(t > T)
        t = T;
    end
    
    %Position/Time
    xr = -(x0+xc)/2 - (x0-xc)/2*cos(2*pi*t/T);
    yr = 0;
    zr = 0.25;
    phir = 0;
    thetar = 0;
    
    xrdot = (61*pi*sin((2*pi*t)/T))/(20*T);
    yrdot = 0;
    
    psir = atan2(yrdot,xrdot);
    psir = 0;
    
    % desired second derivatives
    xrddot = (61*pi^2*cos((2*pi*t)/T))/(10*T^2);
    yrddot = 0;
    
    if(xrdot == 0)
        xrdot = 0.01;
    end
    
    % desired theta derivative
    thetardot = (yrddot - xrddot*tan(thetar))/(xrdot*(1+tan(thetar)^2));

    vr     = xrdot;%sqrt(xrdot^2+yrdot^2);
    omegar = thetardot;
    
    qr = [xr yr zr phir thetar psir]';
    ur = [vr omegar]';
end

== matlab function RobotControl1_640_480/Open-loop control/Vision System/Motion Simulation/kinematic_model ==
  data: u input; q input; qdot output
function qdot = kinematic(u,q)
% Kinematic Model

% q = [x y theta]^T
% qdot = [xdot ydot thetadot]^T
% u = [v omega]^T

qdot = zeros(3,1);

theta = q(3);
qdot = [cos(theta),0;sin(theta),0;0,1]*u; % Eq.(2)

== matlab function RobotControl1_640_480/Open-loop control/PWM Calculation ==
  data: enable input; v input; PWM_L output; omega input; PWM_R output; g1 input; g2 input
function [PWM_L, PWM_R] = PWM(enable, v, omega, g1, g2)
%#codegen

if enable == -1
    v = 0;
    omega = 0;
end

T = 0.422;
vL = v -(T/2)*omega;
vR = v +(T/2)*omega;

%----------------------------------
%Calculations for left wheel motor
if(vL < -1.7)
    PWM_L = 1000;
    
elseif(vL < 0)
    %function for the negative area
    PWM_L = 70.971*vL^3 + 264.6006*vL^2 + 479.6339*vL + 1395.7533;
    
% elseif(vL < 0.04)
%     PWM_L = 1500;
    
elseif(vL < 1.7)
    %function for the positive area
    PWM_L = 45.3547*vL^3 + -181.5969*vL^2 + 411.962*vL + 1590.6833 + g1;

else
    PWM_L = 2000;
    
end

%----------------------------------
%Calculations for right wheel motor
if(vR < -1.7)
    PWM_R = 1000;
    
elseif(vR < 0)
    %function for negative area
    PWM_R = 73.2531*vR^3 + 266.55*vR^2 + 478.8239*vR + 1400.4623 - g2;

% elseif(vR < 0.04)
%     PWM_R = 1500;
    
elseif(vR < 1.7)
    %function for positve area
    PWM_R = 47.0508*vR^3 + -193.9456*vR^2 + 429.0898*vR + 1593.7706;

else
    PWM_R = 2000;
    
end

% v = 1950;
% PWM_L = v;
% PWM_R = v;

== matlab function RobotControl1_640_480/Open-loop control/Camera Servos Function ==
  data: t input; PAN output; TILT output
 function [PAN,TILT] = fcn(t)
%Insert Function for camera servo manipulation here
%By default, this function holds camera servos at their center position (1500 ms)
PAN = 1525;
TILT = 1400;

== matlab function RobotControl1_640_480/Open-loop control/plant/pulse transformer camera ==
  data: PAN input; TILT input; PAN_O output; TILT_O output
function [PAN_O, TILT_O]  = fcn(PAN,TILT)

PAN_O  = uint16(PAN);
TILT_O = uint16(TILT);

== matlab function RobotControl1_640_480/Open-loop control/MATLAB Function ==
  data: t input; v output; omega output
function [v, omega] = fcn(t)
%#codegen
if(t < 24)
    v = 0.1;
    omega = 0;
else
    v = 0;
    omega = 0;
end

== matlab function RobotControl1_640_480/Open-loop control/Vision System/Sensor1/Read_Filter_ConvertTo2D/IMU Data/Command State ==
  data: ID input; count input; run output
function run = fcn(ID,count)

% In this program the signal ID and count will be checked 
% for the reliability of the data.

if count==42
    if ID==20017
        run=1;
    else
        run=0;
    end
else
    run=0;
end

== matlab function RobotControl1_640_480/Open-loop control/plant/pulse transformer1 ==
  data: Left_PWM_I input; Right_PWM_I input; Left_PWM output; Right_PWM output
function [Left_PWM, Right_PWM]  = fcn(Left_PWM_I,Right_PWM_I)
% This block supports an embeddable subset of the MATLAB language.
% Converts output angle and speed value into a pulse width
% The input angle is between +pi/4 and -pi/4  (from limits)
% The speed is between 140 and 0 rps(Hz)

% angle=uint16(angI*16.25*180/pi + 1505.5);
% pw=-0.0002*speedI^3 +0.03*speedI^2 -2.66*speedI +1528;
% throtle = uint16(pw);
% 
Left_PWM  = uint16(Left_PWM_I);
Right_PWM = uint16(Right_PWM_I);

== matlab function RobotControl1_640_480/Open-loop control/Vision System/Sensor1/Read_Filter_ConvertTo2D/IMU Data/State filter ==
  data: roll input; Qf output; rollrate input; acc input; vel input; pos input
function Qf = fcn( roll, rollrate, acc, vel, pos)
% This block supports an embeddable subset of the MATLAB language.
% See the help menu for details. 

% info is extracted from sensor
rol=roll(1);
pit=roll(2);
yaw=roll(3);
rollp=rollrate(1);
pitp=rollrate(2);
yawp=rollrate(3);
lon=pos(1);
lat=pos(2);
alt=pos(3);
vN=vel(1);
vE=vel(2);
vD=vel(3);
ax=acc(1);
ay=acc(2);
az=acc(3);

Qf = [ax;ay;az];

== matlab function RobotControl1_640_480/Status Extraction/Command State ==
  data: ID input; CCS output; byte input
function CCS = fcn(ID, byte)
% This block supports an embeddable subset of the MATLAB language.
% See the help menu for details. 
% outputs the command channel state (CCS) given status output

% first check that have proper status message
% ID = 10 for SSC status info
if ID==10
    if byte==2
        out=1;
    elseif byte==4;
        out=2;
    elseif byte==6
        out=3;
    else
        out=0;
    end
else
    out=4;
end
CCS = out;

== matlab function RobotControl1_640_480/status checker ==
  data: status input; enable output
function enable = s2e(status)
% This block supports an embeddable subset of the MATLAB language.
% See the help menu for details. 
if status==1  
    en = 1;
else
    en = -1;
end

enable=en;

== matlab function RobotControl1_640_480/Open-loop control/plant/Send Serial Packet to Servo Controller And recieve status message from SSC/Embedded MATLAB Function ==
  data: Packed input; CharArray output
function CharArray = fcn(Packed)
%
CharArray = zeros(22,1,'uint8');
CharArray = Packed;
